simulink model "powertrain_myBatt_myMotor"  (R2019a)
settings: Solver=VariableStepAuto  StartTime=0.0  StopTime=1600  FixedStep=.01  RelTol=1e-3
libraries: simulink x5
settings Model: Creator=tdarrah  LastModifiedBy=tdarrah
settings SolverCC: ShapePreserveControl=EnableAll
settings DebuggingCC: ArithmeticOperatorsInVariantConditions=warning

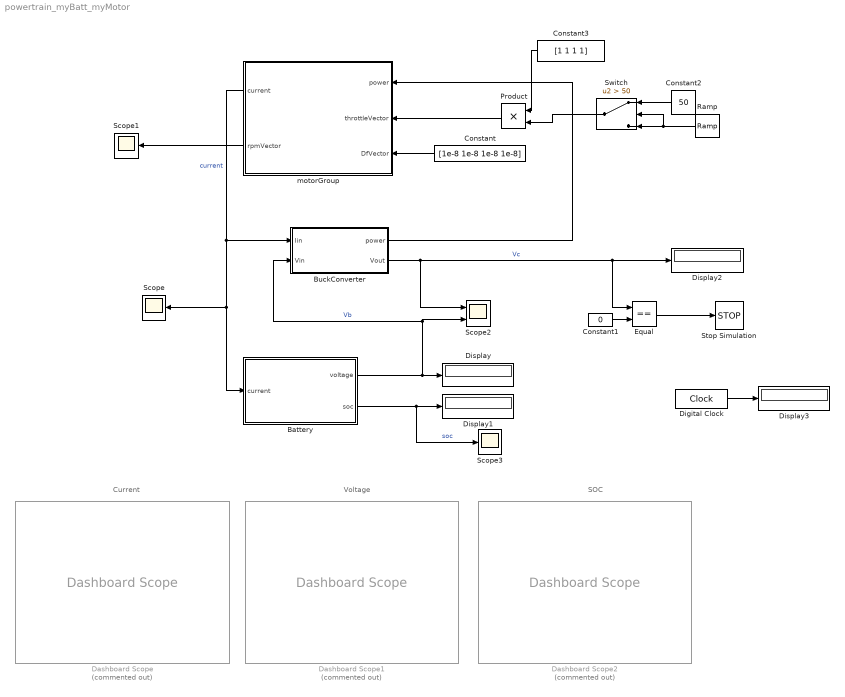
== system powertrain_myBatt_myMotor ==
  note: Current
  note: Voltage
  note: SOC
  Battery : Subsystem
  BuckConverter : Subsystem
  Constant : Constant  Value=[1e-8 1e-8 1e-8 1e-8]
  Constant1 : Constant  Value=0
  Constant2 : Constant  Value=50
  Constant3 : Constant  Value=[1 1 1 1]
  Dashboard Scope : DashboardScope  Commented=on  Ymin=-5  Ymax=10
  Dashboard Scope1 : DashboardScope  Commented=on  Ymin=8  Ymax=13
  Dashboard Scope2 : DashboardScope  Commented=on
  Digital Clock : DigitalClock
      mask Display: disp('Sim Time');
  Display{,1..3} (4 alike) : Display
  Equal : RelationalOperator  Operator===  OutDataTypeStr=boolean  RndMeth=Simplest
  Product : Product
  Ramp : simulink/Sources/Ramp  slope=1  start=0  InitialOutput=0
  Scope : Scope
  Scope1 : Scope
  Scope2 : Scope  NumInputPorts=2
  Scope3 : Scope
  Stop Simulation : Stop
  Switch : Switch  Criteria=u2 > Threshold  Threshold=50
  motorGroup : Subsystem
  wires:
  Battery/1(voltage) -> BuckConverter/2(Vin), Scope2/2, Display/1  "Vb"
  Battery/2(soc) -> Scope3/1, Display1/1  "soc"
  motorGroup/1(current) -> BuckConverter/1(Iin), Battery/1(current), Scope/1  "current"
  BuckConverter/1(power) -> motorGroup/1(power)
  BuckConverter/2(Vout) -> Scope2/1, Equal/1, Display2/1  "Vc"
  Product/1 -> motorGroup/2(throttleVector)
  Constant/1 -> motorGroup/3(DfVector)
  motorGroup/2(rpmVector) -> Scope1/1
  Constant1/1 -> Equal/2
  Equal/1 -> Stop Simulation/1
  Digital Clock/1 -> Display3/1
  Ramp/1 -> Switch/2, Switch/3
  Constant2/1 -> Switch/1
  Constant3/1 -> Product/1
  Switch/1 -> Product/2

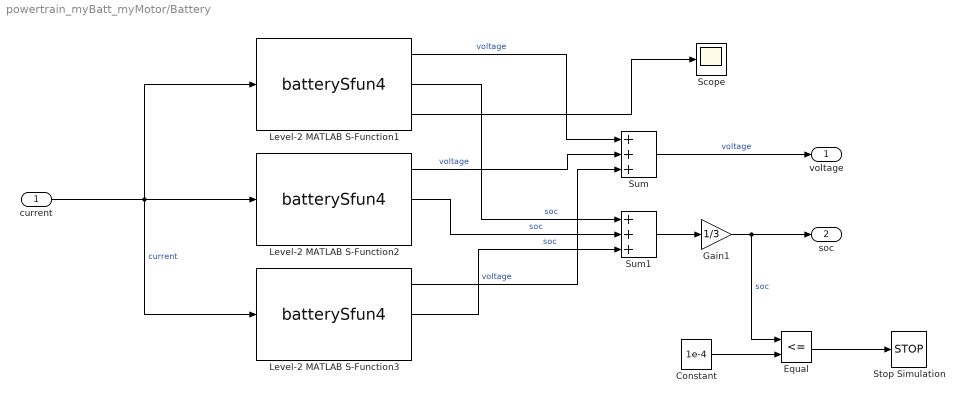
== system powertrain_myBatt_myMotor/Battery ==
  current : Inport
  Constant : Constant  Value=1e-4
  Equal : RelationalOperator  Operator=<=  OutDataTypeStr=boolean  RndMeth=Simplest
  Gain1 : Gain  Gain=1/3
  Level-2 MATLAB S-Function1 : M-S-Function  FunctionName=batterySfun4  Parameters=battery, soc_ocv, .0035
      mask Display:
      | port_label('input', 1, 'current');
      | port_label('output', 1, 'voltage');
      | port_label('output', 2, 'soc');
  Level-2 MATLAB S-Function2 : M-S-Function  FunctionName=batterySfun4  Parameters=battery, soc_ocv, .0035
      mask Display:
      | port_label('input', 1, 'current');
      | port_label('output', 1, 'voltage');
      | port_label('output', 2, 'soc');
  Level-2 MATLAB S-Function3 : M-S-Function  FunctionName=batterySfun4  Parameters=battery, soc_ocv, .0035
      mask Display:
      | port_label('input', 1, 'current');
      | port_label('output', 1, 'voltage');
      | port_label('output', 2, 'soc');
  Scope : Scope
  Stop Simulation : Stop
  Sum : Sum  Inputs=+++
  Sum1 : Sum  Inputs=+++
  voltage : Outport
  soc : Outport  Port=2
  wires:
  Level-2 MATLAB S-Function2/1 -> Sum/2  "voltage"
  Level-2 MATLAB S-Function1/1 -> Sum/1  "voltage"
  Level-2 MATLAB S-Function2/2 -> Sum1/2  "soc"
  Sum1/1 -> Gain1/1
  Gain1/1 -> Equal/1, soc/1  "soc"
  Level-2 MATLAB S-Function1/2 -> Sum1/1  "soc"
  Level-2 MATLAB S-Function3/2 -> Sum1/3  "soc"
  current/1 -> Level-2 MATLAB S-Function3/1, Level-2 MATLAB S-Function1/1, Level-2 MATLAB S-Function2/1  "current"
  Level-2 MATLAB S-Function3/1 -> Sum/3  "voltage"
  Sum/1 -> voltage/1  "voltage"
  Level-2 MATLAB S-Function1/3 -> Scope/1
  Constant/1 -> Equal/2
  Equal/1 -> Stop Simulation/1

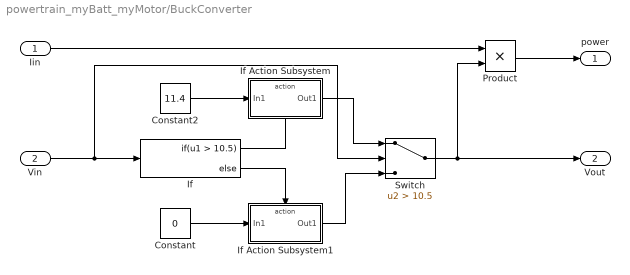
== system powertrain_myBatt_myMotor/BuckConverter ==
  Iin : Inport
  Vin : Inport  Port=2
  Constant : Constant  Value=0
  Constant2 : Constant  Value=11.4
  If : If  IfExpression=u1 > 10.5
  If Action Subsystem : Subsystem  TreatAsAtomicUnit=on
  If Action Subsystem1 : Subsystem  TreatAsAtomicUnit=on
  Product : Product
  Switch : Switch  Criteria=u2 > Threshold  Threshold=10.5
  power : Outport
  Vout : Outport  Port=2
  wires:
  Product/1 -> power/1
  Iin/1 -> Product/1
  If/1 -> If Action Subsystem/Action
  If/2 -> If Action Subsystem1/Action
  Constant/1 -> If Action Subsystem1/1(In1)
  If Action Subsystem/1(Out1) -> Switch/1
  If Action Subsystem1/1(Out1) -> Switch/3
  Constant2/1 -> If Action Subsystem/1(In1)
  Vin/1 -> Switch/2, If/1
  Switch/1 -> Product/2, Vout/1

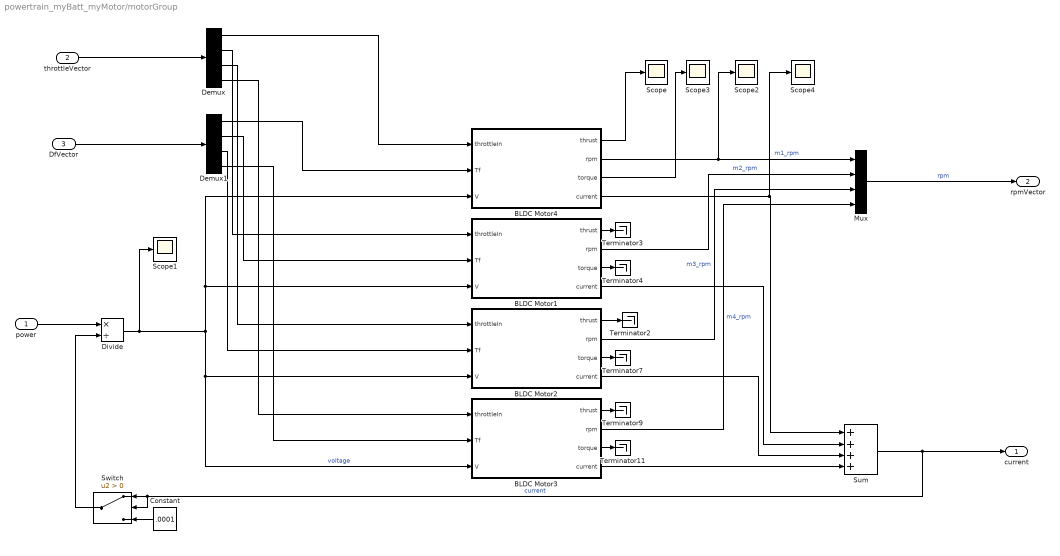
== system powertrain_myBatt_myMotor/motorGroup ==
  power : Inport
  throttleVector : Inport  Port=2  PortDimensions=4
  DfVector : Inport  Port=3  PortDimensions=4
  BLDC Motor1 : Subsystem
  BLDC Motor2 : Subsystem
  BLDC Motor3 : Subsystem
  BLDC Motor4 : Subsystem
  Constant : Constant  Value=.0001
  Demux : Demux
  Demux1 : Demux
  Divide : Product  Inputs=*/
  Mux : Mux
  Scope{,1..4} (5 alike) : Scope
  Sum : Sum  Inputs=++++
  Switch : Switch  Criteria=u2 > Threshold
  Terminator{2..4,7,9,11} (6 alike) : Terminator
  current : Outport
  rpmVector : Outport  Port=2
  wires:
  Demux1/2 -> BLDC Motor1/2(Tf)
  Demux1/4 -> BLDC Motor3/2(Tf)
  Divide/1 -> Scope1/1, BLDC Motor1/3(V), BLDC Motor4/3(V), BLDC Motor3/3(V), BLDC Motor2/3(V)  "voltage"
  Demux1/1 -> BLDC Motor4/2(Tf)
  Sum/1 -> Switch/2, Switch/1, current/1  "current"
  Demux1/3 -> BLDC Motor2/2(Tf)
  BLDC Motor4/4(current) -> Scope4/1, Sum/1
  power/1 -> Divide/1
  Demux/4 -> BLDC Motor3/1(throttleIn)
  Demux/3 -> BLDC Motor2/1(throttleIn)
  Demux/2 -> BLDC Motor1/1(throttleIn)
  Demux/1 -> BLDC Motor4/1(throttleIn)
  throttleVector/1 -> Demux/1
  DfVector/1 -> Demux1/1
  BLDC Motor3/4(current) -> Sum/4
  BLDC Motor2/4(current) -> Sum/3
  BLDC Motor1/4(current) -> Sum/2
  BLDC Motor3/2(rpm) -> Mux/4  "m4_rpm"
  BLDC Motor2/2(rpm) -> Mux/3  "m3_rpm"
  BLDC Motor1/2(rpm) -> Mux/2  "m2_rpm"
  BLDC Motor4/2(rpm) -> Scope2/1, Mux/1  "m1_rpm"
  Mux/1 -> rpmVector/1  "rpm"
  BLDC Motor4/1(thrust) -> Scope/1
  BLDC Motor3/3(torque) -> Terminator11/1
  BLDC Motor4/3(torque) -> Scope3/1
  BLDC Motor1/3(torque) -> Terminator4/1
  BLDC Motor2/3(torque) -> Terminator7/1
  BLDC Motor3/1(thrust) -> Terminator9/1
  BLDC Motor2/1(thrust) -> Terminator2/1
  BLDC Motor1/1(thrust) -> Terminator3/1
  Switch/1 -> Divide/2
  Constant/1 -> Switch/3

== system powertrain_myBatt_myMotor/BuckConverter/If Action Subsystem ==
  In1 : Inport
  Action Port : ActionPort  ActionPortLabel=if(u1 > 10.5)
  Out1 : Outport
  wires:
  In1/1 -> Out1/1

== system powertrain_myBatt_myMotor/BuckConverter/If Action Subsystem1 ==
  In1 : Inport
  Action Port : ActionPort  ActionPortLabel=else
  Out1 : Outport
  wires:
  In1/1 -> Out1/1

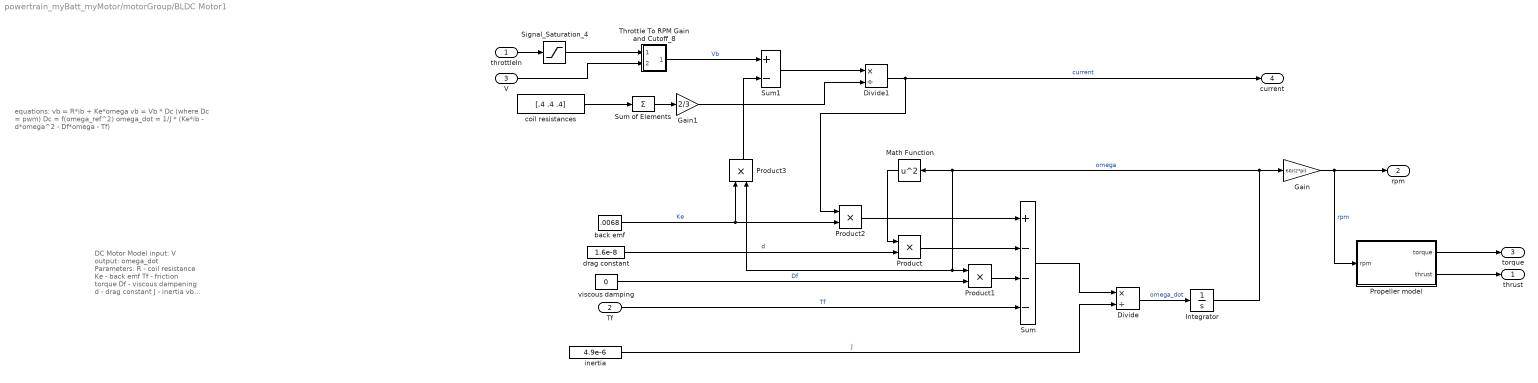
== system powertrain_myBatt_myMotor/motorGroup/BLDC Motor1 ==
  note: DC Motor Model
      |
      | input:
      | V
      |
      | output:
      | omega_dot
      |
      | Parameters:
      | R   - coil resistance
      | Ke - back emf
      | Tf  - friction torque
      | Df  - viscous dampening
      | d   - drag constant
      | J   - inertia
      |
      |
      | vb - average battery voltage
      | ib  - average battery current
  note: equations:
      |
      | vb = R*ib + Ke*omega
      | vb = Vb * Dc  (where Dc = pwm)
      | Dc = f(omega_ref^2)
      |
      | omega_dot = 1/J * (Ke*ib - d*omega^2 - Df*omega - Tf)
  throttleIn : Inport
  Tf : Inport  Port=2
  V : Inport  Port=3
  Divide : Product  Inputs=*/
  Divide1 : Product  Inputs=*/
  Gain : Gain  Gain=60/(2*pi)
  Gain1 : Gain  Gain=2/3
  Integrator : Integrator
  Math Function : Math  Operator=square  SaturateOnIntegerOverflow=on
  Product{,1..3} (4 alike) : Product
  "Propeller model " : MATLAB Function  TreatAsAtomicUnit=on
  Signal_Saturation_4 : Saturate  UpperLimit=100  LowerLimit=0
  Sum : Sum  Inputs=+---
  Sum of Elements : Sum  Inputs=+
  Sum1 : Sum  Inputs=+-
  Throttle To RPM Gain and Cutoff_8 : Subsystem
  back emf : Constant  Value=.0068
  coil resistances : Constant  Value=[.4 .4 .4]
  drag constant : Constant  Value=1.6e-8
  inertia : Constant  Value=4.9e-6
  viscous damping : Constant  Value=0
  thrust : Outport
  rpm : Outport  Port=2
  torque : Outport  Port=3
  current : Outport  Port=4
  wires:
  Divide/1 -> Integrator/1  "omega_dot"
  Integrator/1 -> Math Function/1, Product1/1, Product3/2, Gain/1  "omega"
  Gain/1 -> rpm/1, "Propeller model "/1(rpm)  "rpm"
  inertia/1 -> Divide/2  "J"
  drag constant/1 -> Product/2  "d"
  Math Function/1 -> Product/1
  viscous damping/1 -> Product1/2  "Df"
  Tf/1 -> Sum/4  "Tf"
  back emf/1 -> Product3/1, Product2/2  "Ke"
  Product2/1 -> Sum/1
  Divide1/1 -> Product2/1, current/1  "current"
  V/1 -> Throttle To RPM Gain and Cutoff_8/2(Vs)
  Product3/1 -> Sum1/2
  Sum1/1 -> Divide1/1
  Gain1/1 -> Divide1/2
  "Propeller model "/2(thrust) -> thrust/1
  "Propeller model "/1(torque) -> torque/1
  Product1/1 -> Sum/3
  Product/1 -> Sum/2
  Sum/1 -> Divide/1
  coil resistances/1 -> Sum of Elements/1
  Sum of Elements/1 -> Gain1/1
  throttleIn/1 -> Signal_Saturation_4/1
  Signal_Saturation_4/1 -> Throttle To RPM Gain and Cutoff_8/1(In5)
  Throttle To RPM Gain and Cutoff_8/1(Out5) -> Sum1/1  "Vb"

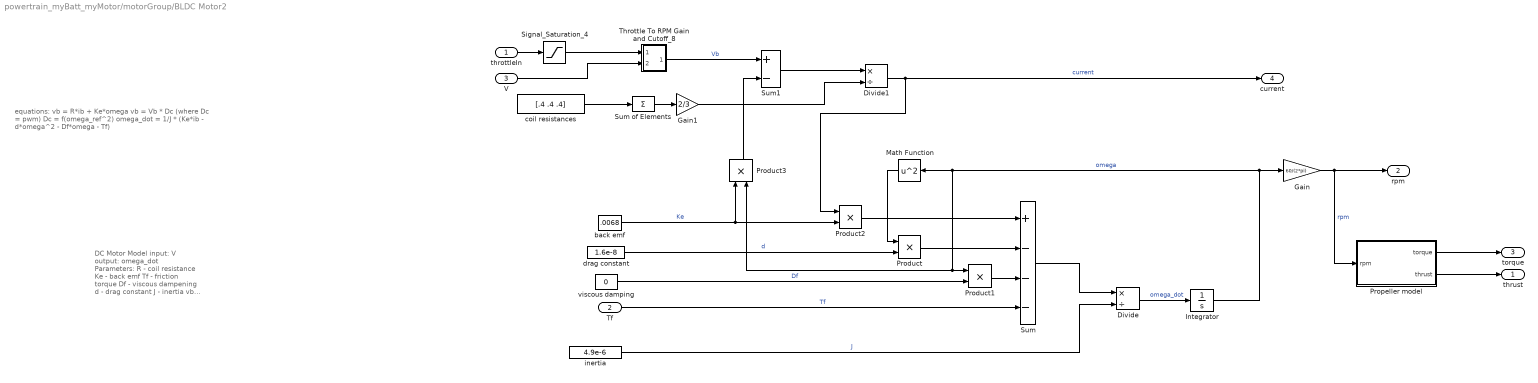
== system powertrain_myBatt_myMotor/motorGroup/BLDC Motor2 ==
  note: DC Motor Model
      |
      | input:
      | V
      |
      | output:
      | omega_dot
      |
      | Parameters:
      | R   - coil resistance
      | Ke - back emf
      | Tf  - friction torque
      | Df  - viscous dampening
      | d   - drag constant
      | J   - inertia
      |
      |
      | vb - average battery voltage
      | ib  - average battery current
  note: equations:
      |
      | vb = R*ib + Ke*omega
      | vb = Vb * Dc  (where Dc = pwm)
      | Dc = f(omega_ref^2)
      |
      | omega_dot = 1/J * (Ke*ib - d*omega^2 - Df*omega - Tf)
  throttleIn : Inport
  Tf : Inport  Port=2
  V : Inport  Port=3
  Divide : Product  Inputs=*/
  Divide1 : Product  Inputs=*/
  Gain : Gain  Gain=60/(2*pi)
  Gain1 : Gain  Gain=2/3
  Integrator : Integrator
  Math Function : Math  Operator=square  SaturateOnIntegerOverflow=on
  Product{,1..3} (4 alike) : Product
  "Propeller model " : MATLAB Function  TreatAsAtomicUnit=on
  Signal_Saturation_4 : Saturate  UpperLimit=100  LowerLimit=0
  Sum : Sum  Inputs=+---
  Sum of Elements : Sum  Inputs=+
  Sum1 : Sum  Inputs=+-
  Throttle To RPM Gain and Cutoff_8 : Subsystem
  back emf : Constant  Value=.0068
  coil resistances : Constant  Value=[.4 .4 .4]
  drag constant : Constant  Value=1.6e-8
  inertia : Constant  Value=4.9e-6
  viscous damping : Constant  Value=0
  thrust : Outport
  rpm : Outport  Port=2
  torque : Outport  Port=3
  current : Outport  Port=4
  wires:
  Divide/1 -> Integrator/1  "omega_dot"
  Integrator/1 -> Math Function/1, Product1/1, Product3/2, Gain/1  "omega"
  Gain/1 -> rpm/1, "Propeller model "/1(rpm)  "rpm"
  inertia/1 -> Divide/2  "J"
  drag constant/1 -> Product/2  "d"
  Math Function/1 -> Product/1
  viscous damping/1 -> Product1/2  "Df"
  Tf/1 -> Sum/4  "Tf"
  back emf/1 -> Product3/1, Product2/2  "Ke"
  Product2/1 -> Sum/1
  Divide1/1 -> Product2/1, current/1  "current"
  V/1 -> Throttle To RPM Gain and Cutoff_8/2(Vs)
  Product3/1 -> Sum1/2
  Sum1/1 -> Divide1/1
  Gain1/1 -> Divide1/2
  "Propeller model "/2(thrust) -> thrust/1
  "Propeller model "/1(torque) -> torque/1
  Product1/1 -> Sum/3
  Product/1 -> Sum/2
  Sum/1 -> Divide/1
  coil resistances/1 -> Sum of Elements/1
  Sum of Elements/1 -> Gain1/1
  throttleIn/1 -> Signal_Saturation_4/1
  Signal_Saturation_4/1 -> Throttle To RPM Gain and Cutoff_8/1(In5)
  Throttle To RPM Gain and Cutoff_8/1(Out5) -> Sum1/1  "Vb"

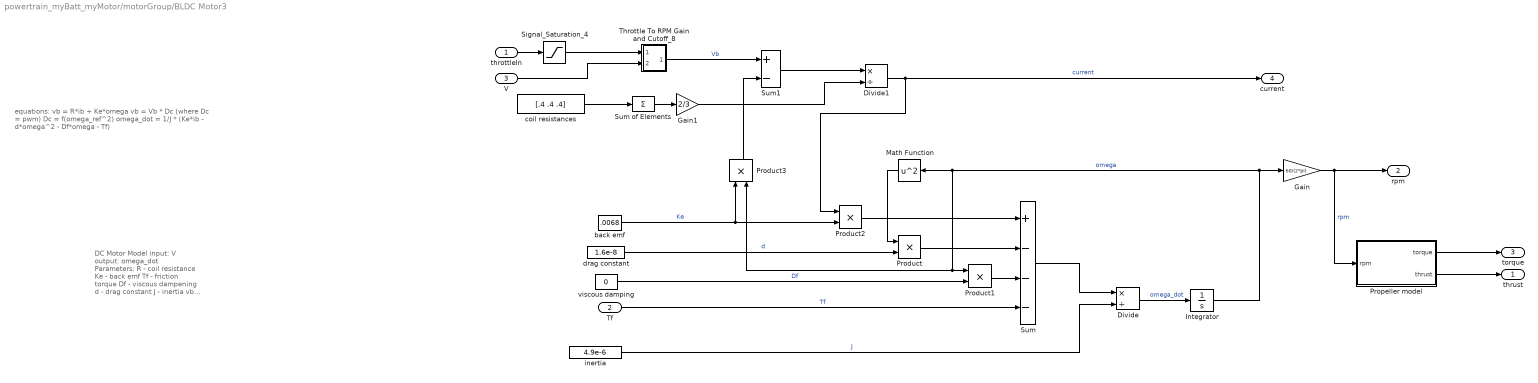
== system powertrain_myBatt_myMotor/motorGroup/BLDC Motor3 ==
  note: DC Motor Model
      |
      | input:
      | V
      |
      | output:
      | omega_dot
      |
      | Parameters:
      | R   - coil resistance
      | Ke - back emf
      | Tf  - friction torque
      | Df  - viscous dampening
      | d   - drag constant
      | J   - inertia
      |
      |
      | vb - average battery voltage
      | ib  - average battery current
  note: equations:
      |
      | vb = R*ib + Ke*omega
      | vb = Vb * Dc  (where Dc = pwm)
      | Dc = f(omega_ref^2)
      |
      | omega_dot = 1/J * (Ke*ib - d*omega^2 - Df*omega - Tf)
  throttleIn : Inport
  Tf : Inport  Port=2
  V : Inport  Port=3
  Divide : Product  Inputs=*/
  Divide1 : Product  Inputs=*/
  Gain : Gain  Gain=60/(2*pi)
  Gain1 : Gain  Gain=2/3
  Integrator : Integrator
  Math Function : Math  Operator=square  SaturateOnIntegerOverflow=on
  Product{,1..3} (4 alike) : Product
  "Propeller model " : MATLAB Function  TreatAsAtomicUnit=on
  Signal_Saturation_4 : Saturate  UpperLimit=100  LowerLimit=0
  Sum : Sum  Inputs=+---
  Sum of Elements : Sum  Inputs=+
  Sum1 : Sum  Inputs=+-
  Throttle To RPM Gain and Cutoff_8 : Subsystem
  back emf : Constant  Value=.0068
  coil resistances : Constant  Value=[.4 .4 .4]
  drag constant : Constant  Value=1.6e-8
  inertia : Constant  Value=4.9e-6
  viscous damping : Constant  Value=0
  thrust : Outport
  rpm : Outport  Port=2
  torque : Outport  Port=3
  current : Outport  Port=4
  wires:
  Divide/1 -> Integrator/1  "omega_dot"
  Integrator/1 -> Math Function/1, Product1/1, Product3/2, Gain/1  "omega"
  Gain/1 -> rpm/1, "Propeller model "/1(rpm)  "rpm"
  inertia/1 -> Divide/2  "J"
  drag constant/1 -> Product/2  "d"
  Math Function/1 -> Product/1
  viscous damping/1 -> Product1/2  "Df"
  Tf/1 -> Sum/4  "Tf"
  back emf/1 -> Product3/1, Product2/2  "Ke"
  Product2/1 -> Sum/1
  Divide1/1 -> Product2/1, current/1  "current"
  V/1 -> Throttle To RPM Gain and Cutoff_8/2(Vs)
  Product3/1 -> Sum1/2
  Sum1/1 -> Divide1/1
  Gain1/1 -> Divide1/2
  "Propeller model "/2(thrust) -> thrust/1
  "Propeller model "/1(torque) -> torque/1
  Product1/1 -> Sum/3
  Product/1 -> Sum/2
  Sum/1 -> Divide/1
  coil resistances/1 -> Sum of Elements/1
  Sum of Elements/1 -> Gain1/1
  throttleIn/1 -> Signal_Saturation_4/1
  Signal_Saturation_4/1 -> Throttle To RPM Gain and Cutoff_8/1(In5)
  Throttle To RPM Gain and Cutoff_8/1(Out5) -> Sum1/1  "Vb"

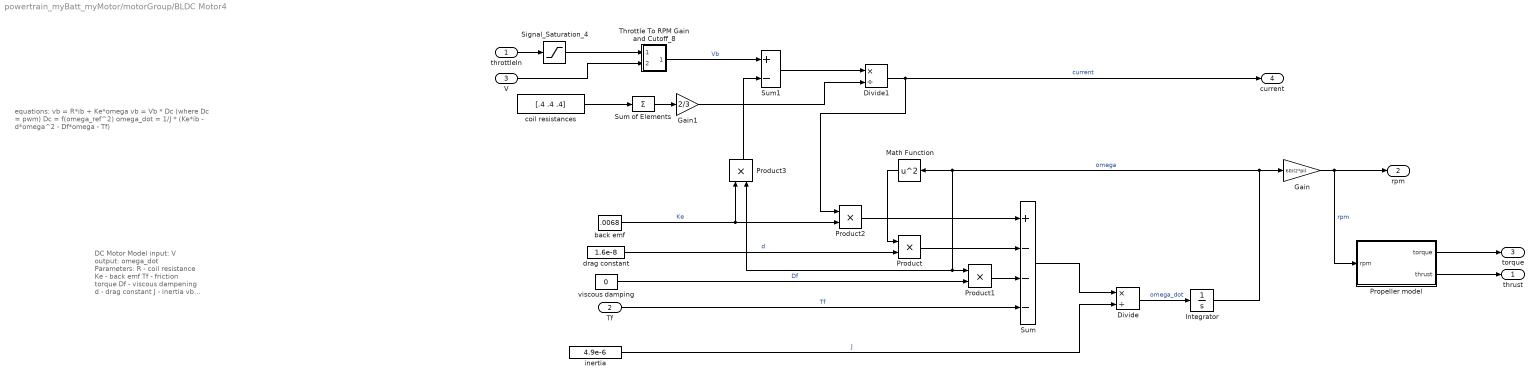
== system powertrain_myBatt_myMotor/motorGroup/BLDC Motor4 ==
  note: DC Motor Model
      |
      | input:
      | V
      |
      | output:
      | omega_dot
      |
      | Parameters:
      | R   - coil resistance
      | Ke - back emf
      | Tf  - friction torque
      | Df  - viscous dampening
      | d   - drag constant
      | J   - inertia
      |
      |
      | vb - average battery voltage
      | ib  - average battery current
  note: equations:
      |
      | vb = R*ib + Ke*omega
      | vb = Vb * Dc  (where Dc = pwm)
      | Dc = f(omega_ref^2)
      |
      | omega_dot = 1/J * (Ke*ib - d*omega^2 - Df*omega - Tf)
  throttleIn : Inport
  Tf : Inport  Port=2
  V : Inport  Port=3
  Divide : Product  Inputs=*/
  Divide1 : Product  Inputs=*/
  Gain : Gain  Gain=60/(2*pi)
  Gain1 : Gain  Gain=2/3
  Integrator : Integrator
  Math Function : Math  Operator=square  SaturateOnIntegerOverflow=on
  Product{,1..3} (4 alike) : Product
  "Propeller model " : MATLAB Function  TreatAsAtomicUnit=on
  Signal_Saturation_4 : Saturate  UpperLimit=100  LowerLimit=0
  Sum : Sum  Inputs=+---
  Sum of Elements : Sum  Inputs=+
  Sum1 : Sum  Inputs=+-
  Throttle To RPM Gain and Cutoff_8 : Subsystem
  back emf : Constant  Value=.0068
  coil resistances : Constant  Value=[.4 .4 .4]
  drag constant : Constant  Value=1.6e-8
  inertia : Constant  Value=4.9e-6
  viscous damping : Constant  Value=0
  thrust : Outport
  rpm : Outport  Port=2
  torque : Outport  Port=3
  current : Outport  Port=4
  wires:
  Divide/1 -> Integrator/1  "omega_dot"
  Integrator/1 -> Math Function/1, Product1/1, Product3/2, Gain/1  "omega"
  Gain/1 -> rpm/1, "Propeller model "/1(rpm)  "rpm"
  inertia/1 -> Divide/2  "J"
  drag constant/1 -> Product/2  "d"
  Math Function/1 -> Product/1
  viscous damping/1 -> Product1/2  "Df"
  Tf/1 -> Sum/4  "Tf"
  back emf/1 -> Product3/1, Product2/2  "Ke"
  Product2/1 -> Sum/1
  Divide1/1 -> Product2/1, current/1  "current"
  V/1 -> Throttle To RPM Gain and Cutoff_8/2(Vs)
  Product3/1 -> Sum1/2
  Sum1/1 -> Divide1/1
  Gain1/1 -> Divide1/2
  "Propeller model "/2(thrust) -> thrust/1
  "Propeller model "/1(torque) -> torque/1
  Product1/1 -> Sum/3
  Product/1 -> Sum/2
  Sum/1 -> Divide/1
  coil resistances/1 -> Sum of Elements/1
  Sum of Elements/1 -> Gain1/1
  throttleIn/1 -> Signal_Saturation_4/1
  Signal_Saturation_4/1 -> Throttle To RPM Gain and Cutoff_8/1(In5)
  Throttle To RPM Gain and Cutoff_8/1(Out5) -> Sum1/1  "Vb"

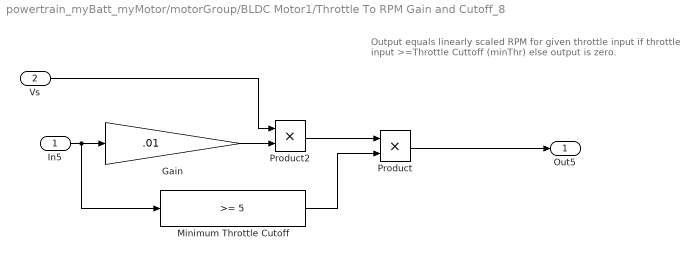
== system powertrain_myBatt_myMotor/motorGroup/BLDC Motor1/Throttle To RPM Gain and Cutoff_8 ==
  note: Output equals linearly scaled RPM
      | for given throttle input if throttle input >=Throttle Cuttoff (minThr)
      | else output is zero.
  In5 : Inport
  Vs : Inport  Port=2
  Gain : Gain  Gain=.01
  Minimum Throttle Cutoff : simulink/Logic and Bit Operations/Compare To Constant  relop=>=  const=5  OutDataTypeStr=uint8
  Product : Product
  Product2 : Product
  Out5 : Outport
  wires:
  Minimum Throttle Cutoff/1 -> Product/2
  Product/1 -> Out5/1
  In5/1 -> Gain/1, Minimum Throttle Cutoff/1
  Gain/1 -> Product2/2
  Product2/1 -> Product/1
  Vs/1 -> Product2/1

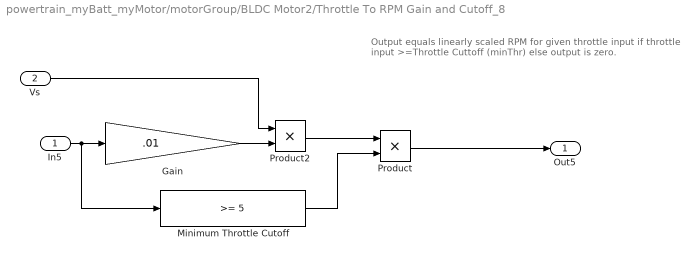
== system powertrain_myBatt_myMotor/motorGroup/BLDC Motor2/Throttle To RPM Gain and Cutoff_8 ==
  note: Output equals linearly scaled RPM
      | for given throttle input if throttle input >=Throttle Cuttoff (minThr)
      | else output is zero.
  In5 : Inport
  Vs : Inport  Port=2
  Gain : Gain  Gain=.01
  Minimum Throttle Cutoff : simulink/Logic and Bit Operations/Compare To Constant  relop=>=  const=5  OutDataTypeStr=uint8
  Product : Product
  Product2 : Product
  Out5 : Outport
  wires:
  Minimum Throttle Cutoff/1 -> Product/2
  Product/1 -> Out5/1
  In5/1 -> Gain/1, Minimum Throttle Cutoff/1
  Gain/1 -> Product2/2
  Product2/1 -> Product/1
  Vs/1 -> Product2/1

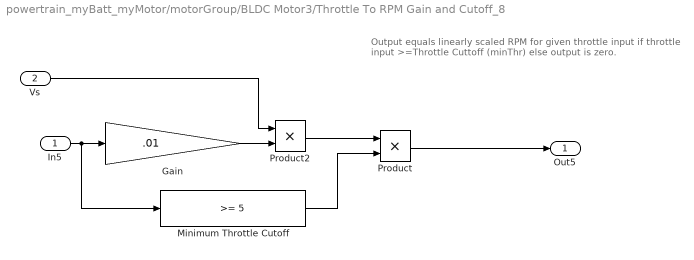
== system powertrain_myBatt_myMotor/motorGroup/BLDC Motor3/Throttle To RPM Gain and Cutoff_8 ==
  note: Output equals linearly scaled RPM
      | for given throttle input if throttle input >=Throttle Cuttoff (minThr)
      | else output is zero.
  In5 : Inport
  Vs : Inport  Port=2
  Gain : Gain  Gain=.01
  Minimum Throttle Cutoff : simulink/Logic and Bit Operations/Compare To Constant  relop=>=  const=5  OutDataTypeStr=uint8
  Product : Product
  Product2 : Product
  Out5 : Outport
  wires:
  Minimum Throttle Cutoff/1 -> Product/2
  Product/1 -> Out5/1
  In5/1 -> Gain/1, Minimum Throttle Cutoff/1
  Gain/1 -> Product2/2
  Product2/1 -> Product/1
  Vs/1 -> Product2/1

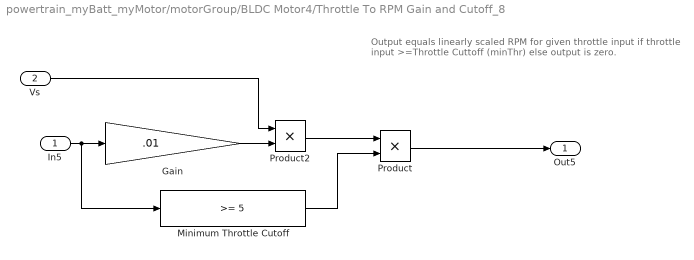
== system powertrain_myBatt_myMotor/motorGroup/BLDC Motor4/Throttle To RPM Gain and Cutoff_8 ==
  note: Output equals linearly scaled RPM
      | for given throttle input if throttle input >=Throttle Cuttoff (minThr)
      | else output is zero.
  In5 : Inport
  Vs : Inport  Port=2
  Gain : Gain  Gain=.01
  Minimum Throttle Cutoff : simulink/Logic and Bit Operations/Compare To Constant  relop=>=  const=5  OutDataTypeStr=uint8
  Product : Product
  Product2 : Product
  Out5 : Outport
  wires:
  Minimum Throttle Cutoff/1 -> Product/2
  Product/1 -> Out5/1
  In5/1 -> Gain/1, Minimum Throttle Cutoff/1
  Gain/1 -> Product2/2
  Product2/1 -> Product/1
  Vs/1 -> Product2/1

== matlab function powertrain_myBatt_myMotor/motorGroup/BLDC Motor4/Propeller model  ==
  data: torque output; rpm input; thrust output
function [torque,thrust] = fcn(rpm)
% angular_velocity in rpm

%coefficient of thrust, empirically derived
coef_t = 2*(10^-15)*rpm^3 - 4*(10^-11)*rpm^2 + 3*(10^-7)*rpm + .1013;
%thrust = coef_t * density of air * velocity^2 * propeller diameter (m) ^4
thrust = coef_t*1.225*(rpm/60)^2*.2^4;
% empirically derived
torque = 4*(10^-14)*rpm^3 +  8*(10^-12)*rpm^2 + 3*(10^-6)*rpm;
end

== matlab function powertrain_myBatt_myMotor/motorGroup/BLDC Motor1/Propeller model  ==
  data: torque output; rpm input; thrust output
function [torque,thrust] = fcn(rpm)
% angular_velocity in rpm

%coefficient of thrust, empirically derived
coef_t = 2*(10^-15)*rpm^3 - 4*(10^-11)*rpm^2 + 3*(10^-7)*rpm + .1013;
%thrust = coef_t * density of air * velocity^2 * propeller diameter (m) ^4
thrust = coef_t*1.225*(rpm/60)^2*.2^4;
% empirically derived
torque = 4*(10^-14)*rpm^3 +  8*(10^-12)*rpm^2 + 3*(10^-6)*rpm;
end

== matlab function powertrain_myBatt_myMotor/motorGroup/BLDC Motor2/Propeller model  ==
  data: torque output; rpm input; thrust output
function [torque,thrust] = fcn(rpm)
% angular_velocity in rpm

%coefficient of thrust, empirically derived
coef_t = 2*(10^-15)*rpm^3 - 4*(10^-11)*rpm^2 + 3*(10^-7)*rpm + .1013;
%thrust = coef_t * density of air * velocity^2 * propeller diameter (m) ^4
thrust = coef_t*1.225*(rpm/60)^2*.2^4;
% empirically derived
torque = 4*(10^-14)*rpm^3 +  8*(10^-12)*rpm^2 + 3*(10^-6)*rpm;
end

== matlab function powertrain_myBatt_myMotor/motorGroup/BLDC Motor3/Propeller model  ==
  data: torque output; rpm input; thrust output
function [torque,thrust] = fcn(rpm)
% angular_velocity in rpm

%coefficient of thrust, empirically derived
coef_t = 2*(10^-15)*rpm^3 - 4*(10^-11)*rpm^2 + 3*(10^-7)*rpm + .1013;
%thrust = coef_t * density of air * velocity^2 * propeller diameter (m) ^4
thrust = coef_t*1.225*(rpm/60)^2*.2^4;
% empirically derived
torque = 4*(10^-14)*rpm^3 +  8*(10^-12)*rpm^2 + 3*(10^-6)*rpm;
end
